simulink model "testPID_YawRotation"  (R2021a)
settings: Solver=VariableStepAuto  StartTime=0.0  StopTime=Torb  RelTol=1e-3
values from neighbouring files (symbols this model uses):
  t0z = 10    [control_1.m]    (also in control_2.m; control_extra2.m)
  tfz = t0z + tz    [control_1.m]    (also in control_2.m; control_extra2.m)
  Tmax = Fmax*Larm    (= 0.00125)    [control_1.m]    (also in control_2.m; control_3.m; control_4.m; control_extra2.m)
libraries: simulink x3, sharedtransform x1
settings Model: DataDictionary=databus.sldd  Creator=Laura  LastModifiedBy=Laura

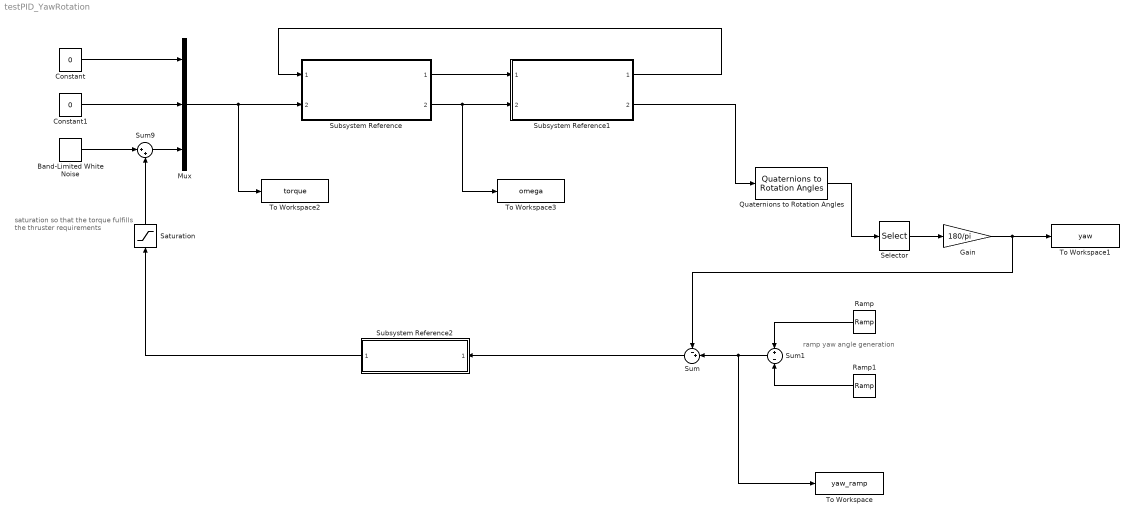
== system testPID_YawRotation ==
  note: ramp yaw angle generation
  note: saturation so that the torque fulfills the thruster requirements
  Band-Limited White Noise : simulink/Sources/Band-Limited White Noise  Cov=[1e-11]  Ts=0.1  seed=[23341]
  Constant : Constant  Value=0
  Constant1 : Constant  Value=0
  Gain : Gain  Gain=180/pi
  Mux : Mux  Inputs=3
  Quaternions to Rotation Angles : sharedtransform/Quaternions to Rotation Angles  rotationOrder=ZYX  aMode=aMode
      settings: SourceProductBaseCode=AE,PW,DR,MT,UV,VE
  Ramp : simulink/Sources/Ramp  slope=45/(tfz-t0z)  start=t0z  InitialOutput=0
  Ramp1 : simulink/Sources/Ramp  slope=45/(tfz-t0z)  start=tfz  InitialOutput=0
  Saturation : Saturate  UpperLimit=Tmax  LowerLimit=-Tmax
  Selector : Selector  InputPortWidth=3  IndexOptions=Index vector (dialog)  Indices=[1]  OutputSizes=1
  Subsystem Reference : Subsystem  ReferencedSubsystem=Dynamics
  Subsystem Reference1 : Subsystem  ReferencedSubsystem=Kinematics
  Subsystem Reference2 : Subsystem  ReferencedSubsystem=PID
  Sum : Sum  Inputs=-+|
  Sum1 : Sum  Inputs=+-
  Sum9 : Sum  Inputs=|++
  To Workspace : ToWorkspace  VariableName=yaw_ramp  SaveFormat=Timeseries  SampleTime=-1
  To Workspace1 : ToWorkspace  VariableName=yaw  SaveFormat=Timeseries  SampleTime=-1
  To Workspace2 : ToWorkspace  VariableName=torque  SaveFormat=Timeseries  SampleTime=-1
  To Workspace3 : ToWorkspace  VariableName=omega  SaveFormat=Timeseries  SampleTime=-1
  wires:
  Subsystem Reference1/1 -> Subsystem Reference/1
  Subsystem Reference1/2 -> Quaternions to Rotation Angles/1
  Subsystem Reference/2 -> To Workspace3/1, Subsystem Reference1/2
  Subsystem Reference/1 -> Subsystem Reference1/1
  Gain/1 -> Sum/1, To Workspace1/1
  Constant/1 -> Mux/1
  Mux/1 -> To Workspace2/1, Subsystem Reference/2
  Constant1/1 -> Mux/2
  Sum9/1 -> Mux/3
  Band-Limited White Noise/1 -> Sum9/1
  Quaternions to Rotation Angles/1 -> Selector/1
  Selector/1 -> Gain/1
  Sum/1 -> Subsystem Reference2/1
  Subsystem Reference2/1 -> Saturation/1
  Saturation/1 -> Sum9/2
  Ramp/1 -> Sum1/1
  Ramp1/1 -> Sum1/2
  Sum1/1 -> To Workspace/1, Sum/2
